simulink model "batteryModel2022a"  (R2022a)
settings: Solver=VariableStepAuto  StartTime=0.0  StopTime=80000  RelTol=1e-3
PreLoadFcn:
  | first_run_this_to_import_nedc_data
  | batteryModel_ini
InitFcn:
  | first_run_this_to_import_nedc_data
  | batteryModel_ini
values from neighbouring files (symbols this model uses):
  Battery =     [BatteryParameters.mat]
  I = [1.29210780767e-28 1.29210780767e-28 1.29210780767e-28 1.29210780767e-28 1.29210780767e-28 1.29210780767e-28 1.29210780767e-28 1.29210780767e-28 1.29210780767e-28 1.29210780767e-28 1.29210780767e-28 4.77614030937 ... (41369 elements, 41369x1)]    [BatteryParameters.mat]
  OCVSOC = [2 2 0.95 1.1 0.95 0.79 1.02 0.92 0.75 0.87]    [BatteryParameters.mat]    (also in OCVSOC.mat)
  Ts = 1    [BatteryParameters.mat]    (also in myFunction.m; test1.m)
undefined symbols (not defined in the file or in its folder): sigbuilder_block
libraries: neural x50, fl_lib x7, nesl_utility x6, dspstat3 x3, simulink x2, sharedTrackingLibrary x2, batteryecm_lib x1, ctrlSharedLib x1
(part 3 of 3)

== matlab function batteryModel2022a/EKF/MATLAB Function1 ==
  data: x output; x input; P input; P output; R0 input; R1 input; R2 input; Tau1 input; Tau2 input; I input; V input; Vocv input; vt output; K output; P1 output; P2 output; x1 output; X1 output; X output; A output
function [x,P,vt,K,P1,P2,x1,X1,X,A]=ukf(x,P, R0, R1, R2, Tau1, Tau2, I, V, Vocv)

Q = [1.0e-5 0;0 1.0e-5];
R = 0.1;
T = 1;

u=[I];

L=numel(x);                                 %numer of states
m=1;                                 %numer of measurements
alpha=1;%1e-3;                                 %default, tunable
ki=0;                                       %default, tunable
beta=2;                                     %default, tunable
kappa=0;%alpha^2*(L+ki)-L;                    %scaling factor
c=L+kappa;                                 %scaling factor
Wm=[kappa/c 0.5/c+zeros(1,2*L)];           %weights for means
Wc=Wm;
Wc(1)=Wc(1)+(1-alpha^2+beta);               %weights for covariance
c=sqrt(c);
[X,A]=sigmas(x,P,c);                            %sigma points around x

[x1,X1,P1,X2]=ut(X,Wm,Wc,L,Q,u,Tau1,Tau2,R0,R1,R2);          %unscented transformation of process

[z1,Z1,P2,Z2]=ut1(X1,Wm,Wc,m,R,u,Vocv,R0);       %unscented transformation of measurments
P12=X2*diag(Wc)*Z2';                        %transformed cross-covariance
K=P12*inv(P2);
vt = z1;
x=x1+K*(V-z1);                              %state update
P=P1-K*P12';                                %covariance update

function [y,Y,P,Y1]=ut(X,Wm,Wc,n,R,u,Tau1,Tau2,R0,R1,R2)

L=size(X,2);
y=zeros(n,1);
Y=zeros(n,L);
etta = 1;
Cq = 5 * 3600;
T=1;
for k=1:L                   
    %Y(:,k)=f(X(:,k));
    Y(1,k) = - etta / Cq * u(1) * T + X(1,k);
    %Y(2,k) = (1 - T/(Tau1)) * X(2,k) + R1/Tau1 * u(1);
    Y(2,k) = R1*(1 - exp(-T/(Tau1)))* u(1) + exp(-T/Tau1) * X(2,k) ;
    y=y+Wm(k)*Y(:,k);       
end
Y1=Y-y(:,ones(1,L));
P=Y1*diag(Wc)*Y1'+R;          

function [y,Y,P,Y1]=ut1(X,Wm,Wc,n,R,u,Vocv,R0)


L=size(X,2);
y=zeros(n,1);
Y=zeros(n,L);
T=1;
for k=1:L                   
    %Y(:,k)=f(X(:,k)); 
    Y(:,k) = Vocv - R0 * u(1) - X(2,k);
    y=y+Wm(k)*Y(:,k);       
end
Y1=Y-y(:,ones(1,L));
P=Y1*diag(Wc)*Y1'+R;          



function [X,A]=sigmas(x,P,c)

A = c*chol(P)';
Y = x(:,ones(1,numel(x)));
X = [x Y+A Y-A];

== matlab function batteryModel2022a/UKF/Simulink Function - State Transition Function/f(x,u) ==
  data: x input; R1 input; R2 input; R3 input; t1 input; t2 input; t3 input; Cq input; I input; xdot output
function xdot = fx(x,R1,R2,R3,t1,t2,t3,Cq,I)
xdot = zeros(size(x));
U1 = x(2);
U2 = x(3);
U3 = x(4);
xdot(1) = -I/(3600*Cq);
xdot(2) = -1/t1*U1 + I/(t1/R1);
xdot(3) = -1/t2*U2 + I/(t2/R2);
xdot(4) = -1/t3*U3 + I/(t3/R3);
xdot(5) = 0;

== matlab function batteryModel2022a/EKF/Simulink Function - State Transition Function/f(x,u) ==
  data: x input; R1 input; R2 input; R3 input; t1 input; t2 input; t3 input; Cq input; I input; xdot output
function xdot = fx(x,R1,R2,R3,t1,t2,t3,Cq,I)
xdot = zeros(size(x));
U1 = x(2);
U2 = x(3);
U3 = x(4);
xdot(1) = -I/(3600*Cq);
xdot(2) = -1/t1*U1 + I/(t1/R1);
xdot(3) = -1/t2*U2 + I/(t2/R2);
xdot(4) = -1/t3*U3 + I/(t3/R3);
xdot(5) = 0;

== matlab function batteryModel2022a/EKF/MATLAB Function ==
  data: V input; SOC_Estimated output; I input; T input; Vt_Estimated output; Vt_Error output; Xk input; Xk1 output; R0 input; R1 input; Tau1 input; OCV input; P_x input; P_x1 output; Q_x input; R_x input; Q_x1 output; R_x1 output; V1 output; KalmanGain_x output; Docv_soc input
function [SOC_Estimated, Vt_Estimated, Vt_Error, Xk1, P_x1, Q_x1,R_x1,V1,KalmanGain_x] = fcn(V, I, T, Xk, R0, R1,Tau1 ,OCV, P_x, Q_x, R_x, Docv_soc)

%comment for AEKF
 Q_x = [1.0e-10 0;0 1.0e-10];
 R_x   = 1;

n_x   = size(Xk,1);

DeltaT = 1;

Qn_rated    = 5 * 3600; % Ah to Amp-seconds

SOC = Xk(1);
V1 = Xk(2);

Tau_1 = Tau1;
    
a1 = exp(-DeltaT/Tau_1);
    
b1 = R1 * (1 - exp(-DeltaT/Tau_1));

    
TerminalVoltage = OCV - R0*I - V1;  

C_x    = [Docv_soc -1];

Error_x   = V - TerminalVoltage;
    
Vt_Estimated = TerminalVoltage;
SOC_Estimated = Xk(1);

Vt_Error = Error_x;

    
    A   = [1 0;
           0 a1];

    B   = [-(DeltaT/Qn_rated); b1];

    Xk   = (A * Xk) + (B * I);
    P_x = (A * P_x * A') + Q_x;
    
    KalmanGain_x = (P_x) * (C_x') * (inv((C_x * P_x * C_x') + (R_x)));
    Xk1 = Xk + (KalmanGain_x * Error_x);
    P_x1 = (eye(n_x,n_x) - (KalmanGain_x * C_x)) * P_x;
    
   
    %adaptive ekf (aekf)
    Q_x1 = KalmanGain_x * Error_x * KalmanGain_x';
    R_x1 = Error_x - C_x * P_x * C_x';



    %y = [SOC_Estimated, Vt_Estimated, Vt_Error, Xk1, P_x1];
